simulink model "MODELE_LIN"  (R2019a)
settings: Solver=VariableStepAuto  StartTime=0.0  StopTime=10.0  RelTol=1e-3
settings Model: Creator=gaul2525  LastModifiedBy=gaul2525

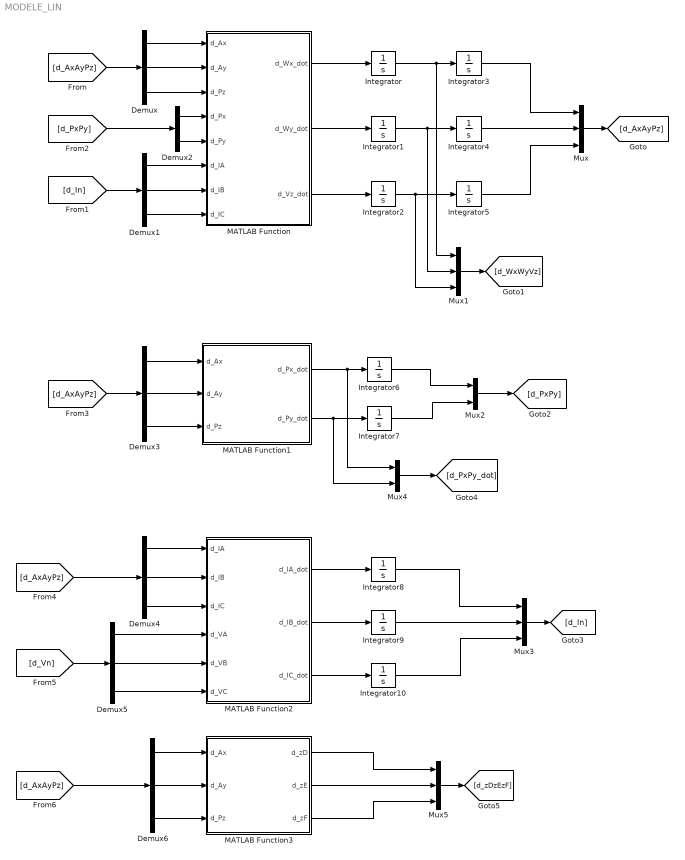
== system MODELE_LIN ==
  Demux{,1,3..6} (6 alike) : Demux  Outputs=3
  Demux2 : Demux  Outputs=2
  Integrator{,1..10} (11 alike) : Integrator
  MATLAB Function : MATLAB Function  TreatAsAtomicUnit=on
  MATLAB Function1 : MATLAB Function  TreatAsAtomicUnit=on
  MATLAB Function2 : MATLAB Function  TreatAsAtomicUnit=on
  MATLAB Function3 : MATLAB Function  TreatAsAtomicUnit=on
  Mux{,1,3,5} (4 alike) : Mux  Inputs=3
  Mux2 : Mux  Inputs=2
  Mux4 : Mux  Inputs=2
  wires:
  MATLAB Function/1(d_Wx_dot) -> Integrator/1
  MATLAB Function/2(d_Wy_dot) -> Integrator1/1
  MATLAB Function/3(d_Vz_dot) -> Integrator2/1
  Integrator4/1 -> Mux/2
  Integrator3/1 -> Mux/1
  Integrator5/1 -> Mux/3
  Mux/1 -> [d_AxAyPz]
  Integrator/1 -> Integrator3/1, Mux1/1
  Integrator1/1 -> Integrator4/1, Mux1/2
  Integrator2/1 -> Integrator5/1, Mux1/3
  Mux1/1 -> [d_WxWyVz]
  MATLAB Function1/1(d_Px_dot) -> Mux4/1, Integrator6/1
  MATLAB Function1/2(d_Py_dot) -> Mux4/2, Integrator7/1
  Integrator6/1 -> Mux2/1
  Integrator7/1 -> Mux2/2
  Mux2/1 -> [d_PxPy]
  MATLAB Function2/1(d_IA_dot) -> Integrator8/1
  MATLAB Function2/2(d_IB_dot) -> Integrator9/1
  MATLAB Function2/3(d_IC_dot) -> Integrator10/1
  Integrator8/1 -> Mux3/1
  Integrator9/1 -> Mux3/2
  Integrator10/1 -> Mux3/3
  Mux3/1 -> [d_In]
  Demux/3 -> MATLAB Function/3(d_Pz)
  Demux/2 -> MATLAB Function/2(d_Ay)
  Demux/1 -> MATLAB Function/1(d_Ax)
  Demux1/1 -> MATLAB Function/6(d_IA)
  Demux1/2 -> MATLAB Function/7(d_IB)
  Demux1/3 -> MATLAB Function/8(d_IC)
  [d_AxAyPz] -> Demux/1
  [d_In] -> Demux1/1
  Demux2/2 -> MATLAB Function/5(d_Py)
  Demux2/1 -> MATLAB Function/4(d_Px)
  [d_PxPy] -> Demux2/1
  Demux3/2 -> MATLAB Function1/2(d_Ay)
  Demux3/1 -> MATLAB Function1/1(d_Ax)
  Demux3/3 -> MATLAB Function1/3(d_Pz)
  [d_AxAyPz] -> Demux3/1
  Demux4/1 -> MATLAB Function2/1(d_IA)
  Demux4/2 -> MATLAB Function2/2(d_IB)
  Demux4/3 -> MATLAB Function2/3(d_IC)
  [d_AxAyPz] -> Demux4/1
  Demux5/2 -> MATLAB Function2/5(d_VB)
  Demux5/1 -> MATLAB Function2/4(d_VA)
  Demux5/3 -> MATLAB Function2/6(d_VC)
  [d_Vn] -> Demux5/1
  Mux4/1 -> [d_PxPy_dot]
  Demux6/2 -> MATLAB Function3/2(d_Ay)
  Demux6/1 -> MATLAB Function3/1(d_Ax)
  [d_AxAyPz] -> Demux6/1
  Demux6/3 -> MATLAB Function3/3(d_Pz)
  MATLAB Function3/2(d_zE) -> Mux5/2
  Mux5/1 -> [d_zDzEzF]
  MATLAB Function3/3(d_zF) -> Mux5/3
  MATLAB Function3/1(d_zD) -> Mux5/1

== matlab function MODELE_LIN/MATLAB Function1 ==
  data: d_Ax input; d_Px_dot output; d_Ay input; d_Pz input; d_Py_dot output
function [d_Px_dot , d_Py_dot] = fcn(d_Ax , d_Ay , d_Pz)

d_Px_dot = 0;
d_Py_dot = 0;

== matlab function MODELE_LIN/MATLAB Function ==
  data: d_Ax input; d_Wx_dot output; d_Ay input; d_Pz input; d_Wy_dot output; d_Px input; d_Py input; d_IA input; d_IB input; d_IC input; d_Vz_dot output
function [d_Wx_dot,d_Wy_dot,d_Vz_dot] = fcn(d_Ax , d_Ay , d_Pz , d_Px , d_Py , d_IA , d_IB , d_IC)

d_Wx_dot = 0;
d_Wy_dot = 0;
d_Vz_dot = 0;

== matlab function MODELE_LIN/MATLAB Function2 ==
  data: d_IA input; d_IA_dot output; d_IB input; d_IC input; d_IB_dot output; d_IC_dot output; d_VA input; d_VB input; d_VC input
function [d_IA_dot , d_IB_dot , d_IC_dot] = fcn(d_IA , d_IB , d_IC , d_VA , d_VB , d_VC)

d_IA_dot = 0;
d_IB_dot = 0;
d_IC_dot = 0;

== matlab function MODELE_LIN/MATLAB Function3 ==
  data: d_Ax input; d_zD output; d_Ay input; d_Pz input; d_zE output; d_zF output
function [d_zD , d_zE , d_zF] = fcn(d_Ax , d_Ay , d_Pz)

d_zD = 0;
d_zE = 0;
d_zF = 0;
